simulink model "KalmanTestes"  (R2021a)
settings: Solver=VariableStepAuto  StartTime=0.0  StopTime=24  RelTol=1e-3
undefined symbols (not defined in the file or in its folder): Continuous, Time
libraries: simulink x2, ctrlSharedLib x1
settings Model: Creator=Pedrus  LastModifiedBy=Pedrus

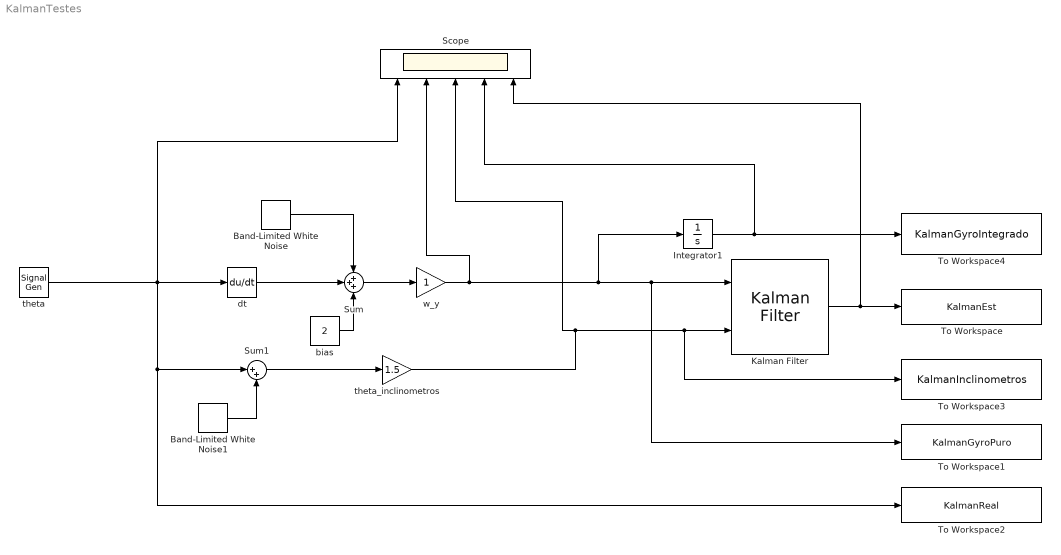
== system KalmanTestes ==
  Band-Limited White Noise : simulink/Sources/Band-Limited White Noise  Cov=[0.6]  Ts=0.1  seed=[23351]
  Band-Limited White Noise1 : simulink/Sources/Band-Limited White Noise  Cov=[0.1]  Ts=0.1  seed=[254651]
  Integrator1 : Integrator
  Kalman Filter : ctrlSharedLib/Kalman Filter  TimeDomain=Continuous-Time  UseCurrentEstimator=on  ModelSource=LTI State-Space Variable  ModelSourceVariable=kalmfpitch  A=0.95  B=1  C=1  D=0  NumberOfStates=1  NumberOfInputs=1  NumberOfOutputs=1  InitialEstimateSource=Dialog  X0=0  P0=10  UseK=off  UseGH=off  NumberOfProcessNoiseInputs=1  G=1  TimeInvariantG=on  H=0  TimeInvariantH=on  Q=1  TimeInvariantQ=on  R=0.25  TimeInvariantR=on  N=0  TimeInvariantN=on  AddInputPort=on  AddEnablePort=off  OutputEstimatedY=off  OutputP=off  Ts=-1
  Scope : Scope  NumInputPorts=5
  Sum : Sum  Inputs=+++
  Sum1 : Sum  Inputs=|++
  To Workspace : ToWorkspace  VariableName=KalmanEst  SaveFormat=Timeseries  SampleTime=-1
  To Workspace1 : ToWorkspace  VariableName=KalmanGyroPuro  SaveFormat=Timeseries  SampleTime=-1
  To Workspace2 : ToWorkspace  VariableName=KalmanReal  SaveFormat=Timeseries  SampleTime=-1
  To Workspace3 : ToWorkspace  VariableName=KalmanInclinometros  SaveFormat=Timeseries  SampleTime=-1
  To Workspace4 : ToWorkspace  VariableName=KalmanGyroIntegrado  SaveFormat=Timeseries  SampleTime=-1
  bias : Constant  Value=2
  dt : Derivative
  theta : SignalGenerator  Amplitude=10  Frequency=0.20
  theta_inclinometros : Gain  Gain=1.5
  w_y : Gain
  wires:
  Kalman Filter/1 -> Scope/5, To Workspace/1
  theta_inclinometros/1 -> Scope/3, Kalman Filter/2, To Workspace3/1
  Integrator1/1 -> Scope/4, To Workspace4/1
  theta/1 -> Scope/1, dt/1, To Workspace2/1, Sum1/1
  Band-Limited White Noise/1 -> Sum/1
  dt/1 -> Sum/2
  Sum/1 -> w_y/1
  w_y/1 -> Kalman Filter/1, To Workspace1/1, Integrator1/1, Scope/2
  bias/1 -> Sum/3
  Sum1/1 -> theta_inclinometros/1
  Band-Limited White Noise1/1 -> Sum1/2
